simulink model "BD_ess_test2"  (Simulink 4.1.1)
settings: Solver=ode1  SolverMode=SingleTasking  StartTime=0.0  StopTime=inf  FixedStep=1  RelTol=1e-3  AbsTol=1e-6
libraries: lib_energy_storage2 x1
settings Model: LastModifiedBy=mokeefe  LimitDataPoints=off  ExtModeTrigMode=oneshot  ExtModeArmWhenConnect=off

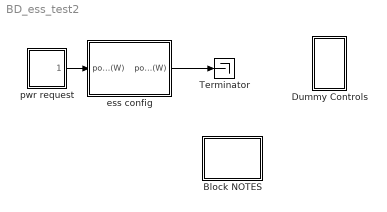
== system BD_ess_test2 ==
  Block NOTES : Subsystem
      settings: RTWFcnNameOpts=Auto  RTWFileNameOpts=Auto
      mask Display: disp('Block\nNOTES')
  Dummy Controls : Subsystem
      settings: RTWFcnNameOpts=Auto  RTWFileNameOpts=Auto
  Terminator : Terminator
  ess config : Subsystem  BlockChoice=energy storage <ess>
      link override energy storage <ess>/From1: GotoTag=essControl
      link override energy storage <ess>/Goto1: GotoTag=essSensors  TagVisibility=global
      link override energy storage <ess>/Goto2: GotoTag=essReqOut  TagVisibility=global
      settings: AttributesFormatString=%<BlockChoice>  TemplateBlock=lib_energy_storage2/ess config  MemberBlocks="Ultracapacitor  System,energy storage <ess>,energy storage <ess> RC,energy storage <ess> nnet,energy storage <ess> Saber,energy storage <ess> fundamental model,energy storage <ess> optima fundamental model"  RTWFcnNameOpts=Auto  RTWFileNameOpts=Auto
  pwr request : Subsystem  mask(Repeating table){@1=ess_pwr_req(:,1), @2=ess_pwr_req(:,2)}
      mask prompts: @1 "Time values:"; @2 "Output values:"
      mask help:
      | Repeating table.
      | Enter values of time and output for first cycle.
      mask init:
      | period = max(@1); t = @1; y = @2;
      settings: RTWFcnNameOpts=Auto  RTWFileNameOpts=Auto
      mask Help: Repeats cycle given in table. Time values should be monotonically increasing.
  wires:
  pwr request/1(out_1) -> ess config/1(power req'd into bus (W))
  ess config/1(power available to bus (W)) -> Terminator/1

== system BD_ess_test2/Block NOTES ==
  note: This model is used with the btry_specs.m script file to determine the discharge power,
      | charge power and energy capacity for a single battery module.
      |  The model is linked to the internal resistance model in the
      | lib_energy_storage.mdl library. (tm:07/24/01)

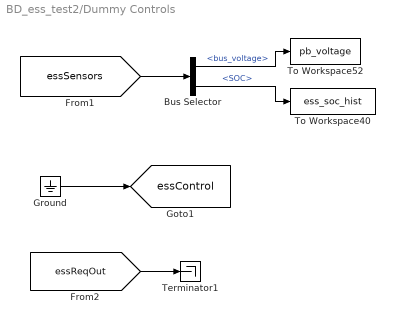
== system BD_ess_test2/Dummy Controls ==
  Bus Selector : BusSelector  OutputSignals=bus_voltage,SOC  MuxedOutput=off
  Ground : Ground
  Terminator1 : Terminator
  To Workspace40 : ToWorkspace  VariableName=ess_soc_hist  SampleTime=-1  SaveFormat=Array
  To Workspace52 : ToWorkspace  VariableName=pb_voltage  SampleTime=-1  SaveFormat=Array
  tag scope: essControl=global
  wires:
  Ground/1 -> [essControl]
  [essSensors] -> Bus Selector/1
  [essReqOut] -> Terminator1/1
  Bus Selector/1 -> To Workspace52/1  "<bus_voltage>"
  Bus Selector/2 -> To Workspace40/1  "<SOC>"

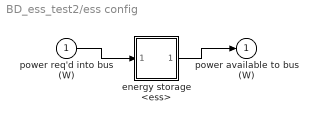
== system BD_ess_test2/ess config ==
  power req'd into bus (W) : Inport  Port=1  LatchInput=off
  energy storage <ess> : Subsystem  AncestorBlock=lib_energy_storage2/energy storage <ess>  mask(Stand-Alone IC Energy Storage System Mask){generalName='ess', logPick=Log Variable, initFileName={}, modCell={}, imgFileName='bdi_ess.jpg'}
      mask prompts: generalName "General Name of this Component [char]"; logPick "Log Variables to Workspace?"; initFileName "Initialization File(s) [cell array of char]"; modCell "Modification Cell [2 column cell array of param and val]"; imgFileName "Icon image file name [char--evaluated]"
      mask init:
      | % initialization via m-file function
      | DB=0; % debug off
      | logFlag=advSACompMaskInit(generalName,logPick,initFileName,modCell,DB);
      settings: RTWFcnNameOpts=Auto  RTWFileNameOpts=Auto
      mask StyleString: edit,popup(Don't Log|Log Variable),edit,edit,edit
      mask Display: image(imread(imgFileName))
  power available to bus (W) : Outport  Port=1
  wires:
  power req'd into bus (W)/1 -> energy storage <ess>/1(power req'd into bus (W))
  energy storage <ess>/1(power available to bus (W)) -> power available to bus (W)/1

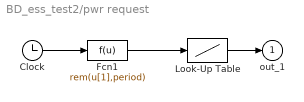
== system BD_ess_test2/pwr request ==
  Clock : Clock
      settings: DisplayTime=off  Decimation=10
  Fcn1 : Fcn  Expr=rem(u[1],period)
  Look-Up Table : Lookup  InputValues=t  OutputValues=y
  out_1 : Outport  Port=1  InitialOutput=0
  wires:
  Look-Up Table/1 -> out_1/1
  Clock/1 -> Fcn1/1
  Fcn1/1 -> Look-Up Table/1

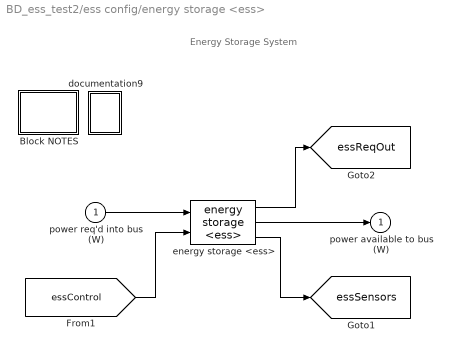
== system BD_ess_test2/ess config/energy storage <ess> ==
  note: Energy Storage System
  power req'd into bus (W) : Inport  Port=1  LatchInput=off
  Block NOTES : Subsystem
      settings: RTWFcnNameOpts=Auto  RTWFileNameOpts=Auto
      mask Display: disp('Block\nNOTES')
  documentation9 : Subsystem
      settings: OpenFcn=web(['file:\\\' which('energy_storage.htm')]);  RTWFcnNameOpts=Auto  RTWFileNameOpts=Auto
      mask Display: image(imread('doc_man.jpg'))
  energy storage <ess> : lib_energy_storage2/Ess Choices/energy storage <ess>
  power available to bus (W) : Outport  Port=1  InitialOutput=0
  tag scope: essReqOut=global, essSensors=global
  wires:
  energy storage <ess>/3 -> [essSensors]
  energy storage <ess>/2 -> power available to bus (W)/1
  energy storage <ess>/1 -> [essReqOut]
  [essControl] -> energy storage <ess>/2
  power req'd into bus (W)/1 -> energy storage <ess>/1

== system BD_ess_test2/ess config/energy storage <ess>/Block NOTES ==
  note: This is a stand-alone version of an energy storage system
      |
      | Several different models are available

== system BD_ess_test2/ess config/energy storage <ess>/documentation9 ==
